simulink model "peregrine_falcon_dive_1"  (R2022a)
settings: Solver=VariableStepAuto  StartTime=0.0  StopTime=10.0  RelTol=1e-3
undefined symbols (not defined in the file): A, Cd, g, m, rho
settings Model: Creator=cc  LastModifiedBy=cc

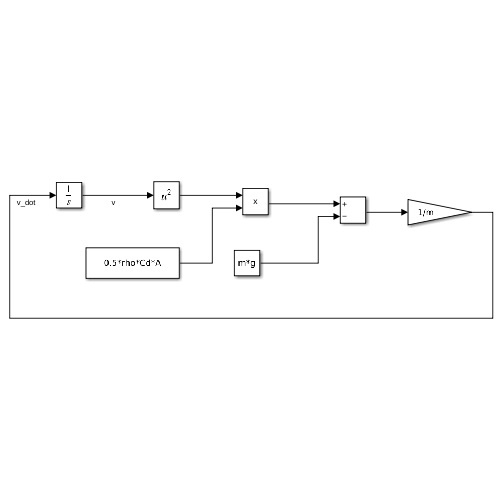
[thumbnail: Simulink's stored preview of the top-level diagram]
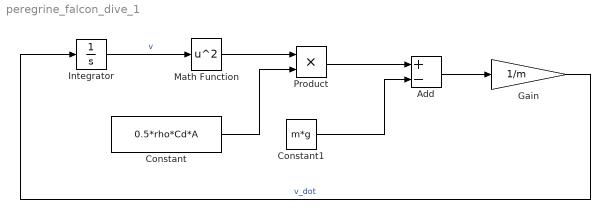
== system peregrine_falcon_dive_1 ==
  Add : Sum  Inputs=+-
  Constant : Constant  Value=0.5*rho*Cd*A
  Constant1 : Constant  Value=m*g
  Gain : Gain  Gain=1/m
  Integrator : Integrator  InitialCondition=-10
  Math Function : Math  Operator=square
  Product : Product
  wires:
  Add/1 -> Gain/1
  Gain/1 -> Integrator/1  "v_dot"
  Constant1/1 -> Add/2
  Integrator/1 -> Math Function/1  "v"
  Math Function/1 -> Product/1
  Constant/1 -> Product/2
  Product/1 -> Add/1
